simulink model "pc_linear_model_with_obs"  (R2020a)
settings: Solver=VariableStepAuto  StartTime=0.0  StopTime=100  RelTol=1e-3
values from neighbouring files (symbols this model uses):
  A_hat = double(subs(A, [mc mp g L d1 d2], [1.5 0.5 9.82 1 .01 .01]))    [pendulum_cart_linear.m]
  B_hat = double(subs(B, [mc L], [1.5 1]))    [pendulum_cart_linear.m]
  C = [1 0 0 0]    [pendulum_cart_linear.m]
  l = acker(A_d', C_d', obs_des_pole_d)    [pendulum_cart_linear.m]
  Ts = .1    (= 0.1)    [pendulum_cart_linear.m]
  x0 = [0 ... (first row only)    [pendulum_cart_linear.m]
undefined symbols (not defined in the file or in its folder): A_d, B_d, C_d, k_lqr_d
settings Model: Creator=mehdikoochak  LastModifiedBy=mehdikoochak

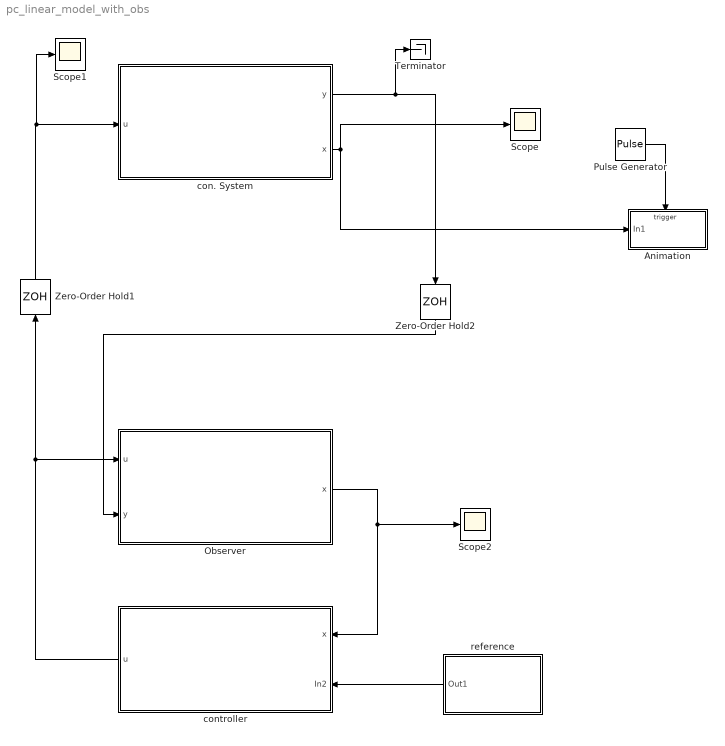
== system pc_linear_model_with_obs ==
  Animation : Subsystem
  Observer : Subsystem
  Pulse Generator : DiscretePulseGenerator  PulseType=Time based  Period=.1  PulseWidth=50
  Scope : Scope
  Scope1 : Scope
  Scope2 : Scope
  Terminator : Terminator
  Zero-Order Hold1 : ZeroOrderHold  SampleTime=Ts
  Zero-Order Hold2 : ZeroOrderHold  SampleTime=Ts
  con. System : Subsystem
  controller : Subsystem
  reference : Subsystem
  wires:
  con. System/1(y) -> Zero-Order Hold2/1, Terminator/1
  con. System/2(x) -> Animation/1(In1), Scope/1
  controller/1(u) -> Observer/1(u), Zero-Order Hold1/1
  Zero-Order Hold1/1 -> Scope1/1, con. System/1(u)
  Observer/1(x) -> Scope2/1, controller/1(x)
  Zero-Order Hold2/1 -> Observer/2(y)
  Pulse Generator/1 -> Animation/Trigger
  reference/1(Out1) -> controller/2(In2)

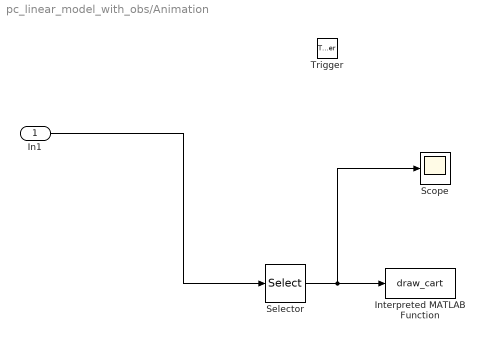
== system pc_linear_model_with_obs/Animation ==
  In1 : Inport
  Trigger : TriggerPort  VariantControl=Variant  PortDimensions=1
  Interpreted MATLAB Function : MATLABFcn  MATLABFcn=draw_cart  OutputDimensions=0
  Scope : Scope
  Selector : Selector  InputPortWidth=4  IndexOptions=Index vector (dialog)  Indices=[1 2]  OutputSizes=1
  wires:
  In1/1 -> Selector/1
  Selector/1 -> Scope/1, Interpreted MATLAB Function/1

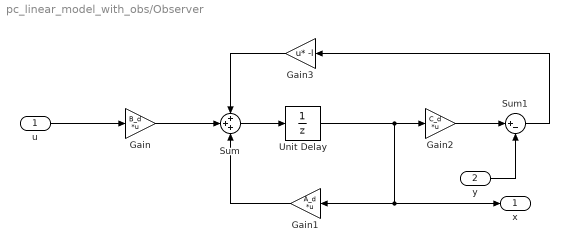
== system pc_linear_model_with_obs/Observer ==
  u : Inport
  y : Inport  Port=2
  Gain : Gain  Gain=B_d  Multiplication=Matrix(K*u)
  Gain1 : Gain  Gain=A_d  Multiplication=Matrix(K*u)
  Gain2 : Gain  Gain=C_d  Multiplication=Matrix(K*u)
  Gain3 : Gain  Gain=-l  Multiplication=Matrix(u*K)
  Sum : Sum  Inputs=+++
  Sum1 : Sum  Inputs=|+-
  Unit Delay : UnitDelay  SampleTime=-1  HasFrameUpgradeWarning=on
  x : Outport
  wires:
  Gain2/1 -> Sum1/1
  Sum/1 -> Unit Delay/1
  u/1 -> Gain/1
  Unit Delay/1 -> x/1, Gain1/1, Gain2/1
  y/1 -> Sum1/2
  Gain1/1 -> Sum/3
  Gain/1 -> Sum/2
  Gain3/1 -> Sum/1
  Sum1/1 -> Gain3/1

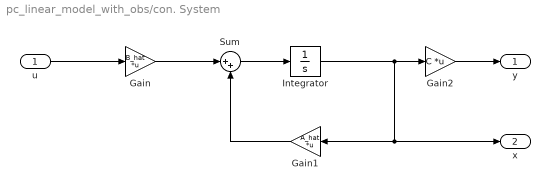
== system pc_linear_model_with_obs/con. System ==
  u : Inport
  Gain : Gain  Gain=B_hat  Multiplication=Matrix(K*u)
  Gain1 : Gain  Gain=A_hat  Multiplication=Matrix(K*u)
  Gain2 : Gain  Gain=C  Multiplication=Matrix(K*u)
  Integrator : Integrator  InitialCondition=x0
  Sum : Sum  Inputs=|++
  y : Outport
  x : Outport  Port=2
  wires:
  Gain2/1 -> y/1
  Gain/1 -> Sum/1
  Sum/1 -> Integrator/1
  u/1 -> Gain/1
  Gain1/1 -> Sum/2
  Integrator/1 -> x/1, Gain1/1, Gain2/1

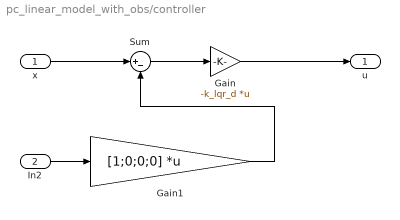
== system pc_linear_model_with_obs/controller ==
  x : Inport
  In2 : Inport  Port=2
  Gain : Gain  Gain=-k_lqr_d  Multiplication=Matrix(K*u)
  Gain1 : Gain  Gain=[1;0;0;0]  Multiplication=Matrix(K*u)
  Sum : Sum  Inputs=|+-
  u : Outport
  wires:
  Gain/1 -> u/1
  x/1 -> Sum/1
  Sum/1 -> Gain/1
  In2/1 -> Gain1/1
  Gain1/1 -> Sum/2

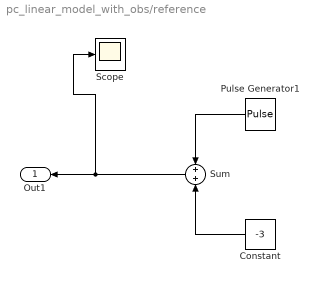
== system pc_linear_model_with_obs/reference ==
  Constant : Constant  Value=-3
  Pulse Generator1 : DiscretePulseGenerator  PulseType=Time based  Amplitude=3  Period=15  PulseWidth=50
  Scope : Scope
  Sum : Sum
  Out1 : Outport
  wires:
  Sum/1 -> Scope/1, Out1/1
  Pulse Generator1/1 -> Sum/1
  Constant/1 -> Sum/2
